simulink model "Part8_2"  (R2021a)
settings: Solver=VariableStepAuto  StartTime=0.0  StopTime=10.0  RelTol=1e-3
undefined symbols (not defined in the file): A, B, C, Disturbance, k, ka
settings Model: Creator=ASUS  LastModifiedBy=ASUS

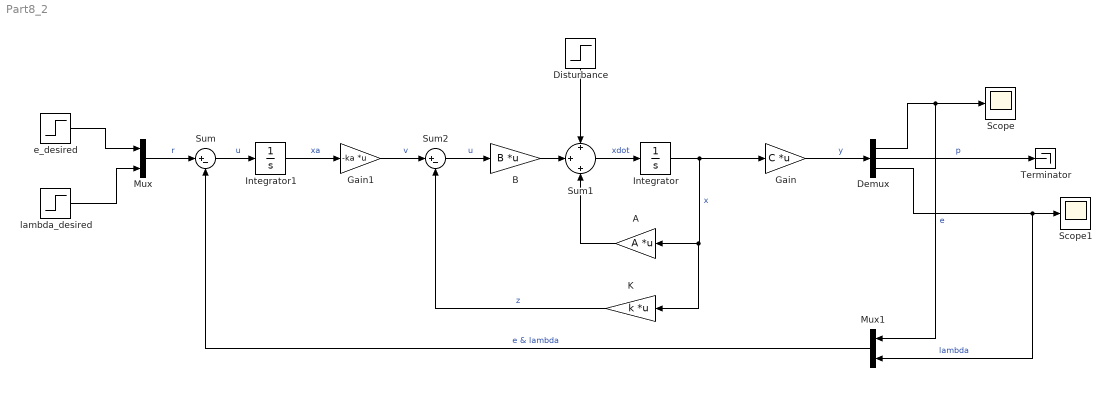
== system Part8_2 ==
  A : Gain  Gain=A  Multiplication=Matrix(K*u)
  B : Gain  Gain=B  Multiplication=Matrix(K*u)
  Demux : Demux  Outputs=3
  Disturbance : Step  Time=0  After=Disturbance  SampleTime=0
  Gain : Gain  Gain=C  Multiplication=Matrix(K*u)
  Gain1 : Gain  Gain=-ka  Multiplication=Matrix(K*u)
  Integrator : Integrator
  Integrator1 : Integrator
  K : Gain  Gain=k  Multiplication=Matrix(K*u)
  Mux : Mux  Inputs=2
  Mux1 : Mux  Inputs=2
  Scope : Scope
  Scope1 : Scope
  Sum : Sum  Inputs=|+-
  Sum1 : Sum  Inputs=+|+|+
  Sum2 : Sum  Inputs=|+-
  Terminator : Terminator
  e_desired : Step  Time=0  After=0.03  SampleTime=0
  lambda_desired : Step  Time=0  After=0.05  SampleTime=0
  wires:
  Demux/2 -> Terminator/1  "p"
  Mux1/1 -> Sum/2  "e & lambda"
  Demux/3 -> Mux1/2, Scope1/1  "lambda"
  e_desired/1 -> Mux/1
  Gain1/1 -> Sum2/1  "v"
  A/1 -> Sum1/3
  lambda_desired/1 -> Mux/2
  Sum1/1 -> Integrator/1  "xdot"
  Sum2/1 -> B/1  "u"
  Integrator/1 -> K/1, A/1, Gain/1  "x"
  Demux/1 -> Mux1/1, Scope/1  "e"
  Gain/1 -> Demux/1  "y"
  B/1 -> Sum1/2
  Integrator1/1 -> Gain1/1  "xa"
  Sum/1 -> Integrator1/1  "u"
  K/1 -> Sum2/2  "z"
  Mux/1 -> Sum/1  "r"
  Disturbance/1 -> Sum1/1
